simulink model "fec_ber_hw"  (R2020b)
settings: Solver=FixedStepDiscrete  StartTime=0.0  StopTime=T/2  RelTol=1e-3
values from neighbouring files (symbols this model uses):
  aximm_awgn_reset = 0    [setup.m]
  aximm_bit_count_reset = 0    [setup.m]
  aximm_bits = n_blocks * k    (= 3200)    [setup.m]
  aximm_ctrl_word_dec = 0    [setup.m]
  aximm_ctrl_word_enc = 0    [setup.m]
  aximm_enable = 1    [setup.m]
  aximm_length = k * n_blocks    (= 3200)    [setup.m]
  aximm_length_dec = n    (= 160)    [setup.m]
  aximm_length_enc = k    (= 80)    [setup.m]
  aximm_llr_mag_reset = 0    [setup.m]
  aximm_llr_scale = (1/noise_var) * llr_scale    (= 1000)    [setup.m]
  aximm_load_dec = 1    [setup.m]
  aximm_load_enc = 1    [setup.m]
  aximm_noise_std = sqrt(noise_var)    [setup.m]
  aximm_reset = 0    [setup.m]
  d = sqrt(-2*log([0:1/4095:1]))    [setup.m]
  fs = 160e6    (= 160000000)    [setup.m]
  llr_scale = 7.75/7.75    (= 1)    [setup.m]
libraries: simulink x450, hdlsllib x190, commseqgen3 x20, dspsigops x17, lib_rfsoc_fec x5, commblkcod2 x3
(part 1 of 22)
settings Model: SimulationMode=accelerator  Creator=ckb13136  LastModifiedBy=ckb13136
settings OptimizationCC: BlockReduction=off  ConditionallyExecuteInputs=off  DefaultParameterBehavior=Inlined
settings DebuggingCC: AlgebraicLoopMsg=error  SingleTaskRateTransMsg=error
settings HardwareCC: ProdBitPerPointer=32  ProdBitPerSizeT=32  ProdBitPerPtrDiffT=32  ProdLargestAtomicFloat=None  ProdIntDivRoundTo=Undefined  ProdEndianess=Unspecified  ProdWordSize=32  ProdHWDeviceType=ASIC/FPGA->ASIC/FPGA  TargetBitPerPointer=64  TargetBitPerSizeT=64  TargetBitPerPtrDiffT=64  TargetLongLongMode=on  TargetIntDivRoundTo=Zero  TargetEndianess=LittleEndian  TargetWordSize=64  TargetHWDeviceType=Custom Processor->MATLAB Host Computer  ProdEqTarget=off

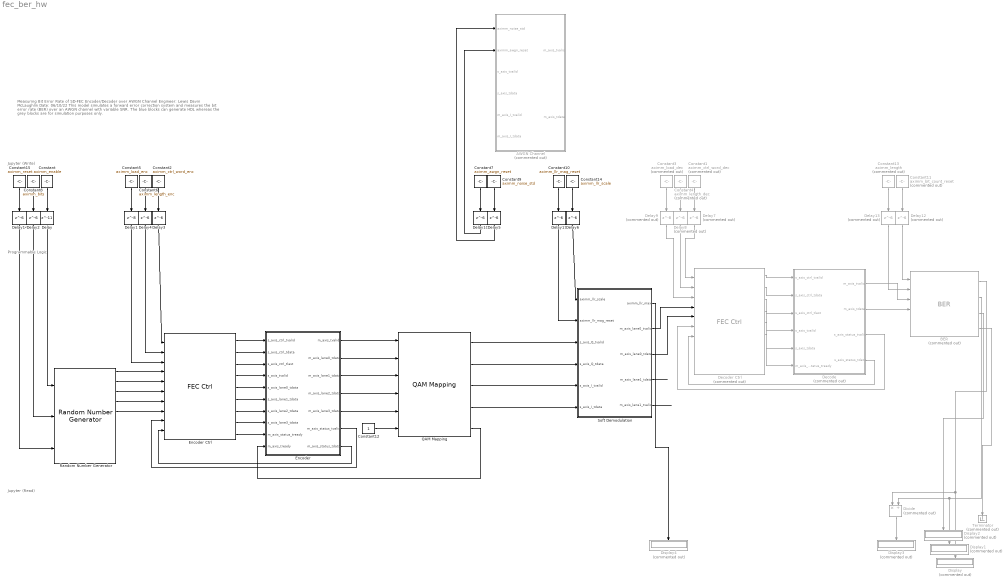
== system fec_ber_hw ==
  note: Measuring Bit Error Rate of SD-FEC Encoder/Decoder over AWGN Channel
      | Engineer: Lewis Davin McLaughlin
      | Date: 06/10/22
      |
      | This model simulates a forward error correction system and measures the bit error rate (BER) over an AWGN channel with variable SNR. The blue blocks can generate HDL whereas the grey blocks are for simulation purposes only.
  note: Jupyter (Write)
  note: Programmable Logic
  note: Jupyter (Read)
  AWGN Channel : Subsystem  Commented=on  AncestorBlock=lib_rfsoc_fec/AWGN Channel  TreatAsAtomicUnit=on
  BER : lib_rfsoc_fec/BER  Commented=on  SystemSampleTime=-1  VariantActivationTime=update diagram  Latency=0  AutoFrameSizeCalculation=off
  Constant : Constant  Value=aximm_enable  OutDataTypeStr=uint32  SampleTime=1/fs
  Constant1 : Constant  Commented=on  Value=aximm_ctrl_word_dec  OutDataTypeStr=uint32  SampleTime=1/(fs*16)
  Constant10 : Constant  Value=aximm_llr_mag_reset  OutDataTypeStr=uint32  SampleTime=1/(fs*2)
  Constant11 : Constant  Commented=on  Value=aximm_bit_count_reset  OutDataTypeStr=uint32  SampleTime=1/(fs*16)
  Constant12 : Constant  OutDataTypeStr=boolean  SampleTime=1/(2*fs)
  Constant13 : Constant  Commented=on  Value=aximm_length  OutDataTypeStr=uint32  SampleTime=1/(fs*16)
  Constant14 : Constant  Value=aximm_llr_scale  OutDataTypeStr=fixdt(0,32,22)  SampleTime=1/(fs*2)
  Constant15 : Constant  Value=aximm_reset  OutDataTypeStr=uint32  SampleTime=1/fs
  Constant2 : Constant  Value=aximm_ctrl_word_enc  OutDataTypeStr=uint32  SampleTime=1/fs
  Constant3 : Constant  Commented=on  Value=aximm_load_dec  OutDataTypeStr=uint32  SampleTime=1/(fs*16)
  Constant4 : Constant  Commented=on  Value=aximm_length_dec  OutDataTypeStr=uint32  SampleTime=1/(fs*16)
  Constant5 : Constant  Value=aximm_load_enc  OutDataTypeStr=uint32  SampleTime=1/fs
  Constant6 : Constant  Value=aximm_length_enc  OutDataTypeStr=uint32  SampleTime=1/fs
  Constant7 : Constant  Value=aximm_awgn_reset  OutDataTypeStr=uint32  SampleTime=1/(fs*2)
  Constant8 : Constant  Value=aximm_bits  OutDataTypeStr=uint32  SampleTime=1/fs
  Constant9 : Constant  Value=aximm_noise_std  OutDataTypeStr=fixdt(0,32,30)  SampleTime=1/(fs*2)
  Decode : Subsystem  Commented=on
  Decoder Ctrl : lib_rfsoc_fec/FEC Ctrl  Commented=on  SystemSampleTime=-1  VariantActivationTime=update diagram  Latency=0  AutoFrameSizeCalculation=off
  Delay : Delay  DelayLength=11
  Delay1 : Delay  DelayLength=8
  Delay{2..6,10..11,14} (8 alike) : Delay  DelayLength=6
  Delay{7..8,12..13} (4 alike) : Delay  Commented=on  DelayLength=6
  Delay9 : Delay  Commented=on  DelayLength=8
  Display{,1..4} (5 alike) : Display  Commented=on
  Divide : Product  Commented=on  Inputs=*/
  Encoder : Subsystem
  Encoder Ctrl : lib_rfsoc_fec/FEC Ctrl  SystemSampleTime=-1  VariantActivationTime=update diagram  Latency=0  AutoFrameSizeCalculation=off
  QAM Mapping : lib_rfsoc_fec/QAM Mapping  SystemSampleTime=-1  VariantActivationTime=update diagram  Latency=0  AutoFrameSizeCalculation=off
  Random Number Generator : lib_rfsoc_fec/Random Number Generator  SystemSampleTime=-1  VariantActivationTime=update diagram  Latency=0  AutoFrameSizeCalculation=off
  Soft Demodulation : Subsystem  AncestorBlock=lib_rfsoc_fec/Soft Demodulation  TreatAsAtomicUnit=on
  Terminator : Terminator  Commented=on
  wires:
  BER/3 -> Display2/1
  Decode/4(s_axis_status_tdata) -> Decoder Ctrl/7
  Soft Demodulation/1(aximm_llr_max) -> Display4/1
  Constant6/1 -> Delay4/1
  Constant3/1 -> Delay9/1
  Decode/3(s_axis_status_tvalid) -> Decoder Ctrl/6
  Constant7/1 -> Delay10/1
  Encoder Ctrl/2 -> Encoder/2(s_axis_ctrl_tdata)
  Decoder Ctrl/6 -> Decode/6(m_axis_status_tready)
  Constant12/1 -> QAM Mapping/6
  Constant4/1 -> Delay8/1
  Encoder Ctrl/6 -> Encoder/6(s_axis_lane1_tdata)
  Constant/1 -> Delay/1
  Delay11/1 -> Soft Demodulation/2(aximm_llr_mag_reset)
  Constant10/1 -> Delay11/1
  Delay9/1 -> Decoder Ctrl/3
  Delay10/1 -> AWGN Channel/2(aximm_awgn_reset)
  Delay/1 -> Random Number Generator/1
  Delay4/1 -> Encoder Ctrl/2
  Delay2/1 -> Random Number Generator/2
  BER/1 -> Divide/1, Display/1
  Soft Demodulation/2(m_axis_lane0_tvalid) -> Decoder Ctrl/4
  Delay12/1 -> BER/1
  Constant11/1 -> Delay12/1
  BER/2 -> Divide/2, Display1/1
  Encoder Ctrl/5 -> Encoder/5(s_axis_lane0_tdata)
  Decoder Ctrl/4 -> Decode/4(s_axis_tvalid)
  Delay8/1 -> Decoder Ctrl/2
  Constant2/1 -> Delay3/1
  Delay7/1 -> Decoder Ctrl/1
  Constant9/1 -> Delay5/1
  Decode/1(m_axis_tvalid) -> BER/3
  Delay1/1 -> Encoder Ctrl/3
  Delay3/1 -> Encoder Ctrl/1
  Decode/2(m_axis_tdata) -> BER/4
  Decoder Ctrl/2 -> Decode/2(s_axis_ctrl_tdata)
  Encoder Ctrl/3 -> Encoder/3(s_axis_ctrl_tlast)
  Decoder Ctrl/3 -> Decode/3(s_axis_ctrl_tlast)
  Divide/1 -> Display3/1
  Encoder/1(m_axis_tvalid) -> QAM Mapping/1
  Delay6/1 -> Soft Demodulation/1(aximm_llr_scale)
  Encoder Ctrl/4 -> Encoder/4(s_axis_tvalid)
  Encoder/7(m_axis_status_tdata) -> Encoder Ctrl/10
  Delay5/1 -> AWGN Channel/1(aximm_noise_std)
  Encoder/2(m_axis_lane0_tdata) -> QAM Mapping/2
  Encoder/6(m_axis_status_tvalid) -> Encoder Ctrl/9
  Decoder Ctrl/1 -> Decode/1(s_axis_ctrl_tvalid)
  Constant14/1 -> Delay6/1
  Decoder Ctrl/5 -> Decode/5(s_axis_tdata)
  Constant8/1 -> Delay2/1
  Encoder Ctrl/1 -> Encoder/1(s_axis_ctrl_tvalid)
  Constant1/1 -> Delay7/1
  Soft Demodulation/3(m_axis_lane0_tdata) -> Decoder Ctrl/5
  Constant5/1 -> Delay1/1
  BER/4 -> Terminator/1
  Constant13/1 -> Delay13/1
  Delay13/1 -> BER/2
  Delay14/1 -> Random Number Generator/3
  Constant15/1 -> Delay14/1
  QAM Mapping/5 -> Encoder/10(m_axis_tready)
  Random Number Generator/3 -> Encoder Ctrl/6
  Random Number Generator/4 -> Encoder Ctrl/7
  Random Number Generator/2 -> Encoder Ctrl/5
  Random Number Generator/1 -> Encoder Ctrl/4
  Random Number Generator/5 -> Encoder Ctrl/8
  Encoder Ctrl/7 -> Encoder/7(s_axis_lane2_tdata)
  Encoder Ctrl/8 -> Encoder/8(s_axis_lane3_tdata)
  Encoder Ctrl/9 -> Encoder/9(m_axis_status_tready)
  Encoder/3(m_axis_lane1_tdata) -> QAM Mapping/3
  Encoder/4(m_axis_lane2_tdata) -> QAM Mapping/4
  Encoder/5(m_axis_lane3_tdata) -> QAM Mapping/5
  QAM Mapping/1 -> Soft Demodulation/3(s_axis_Q_tvalid)
  QAM Mapping/2 -> Soft Demodulation/4(s_axis_Q_tdata)
  QAM Mapping/3 -> Soft Demodulation/5(s_axis_I_tvalid)
  QAM Mapping/4 -> Soft Demodulation/6(s_axis_I_tdata)
  Soft Demodulation/4(m_axis_lane1_tdata) -> ?
  Soft Demodulation/5(m_axis_lane1_tvalid) -> ?

== system fec_ber_hw/AWGN Channel ==
  aximm_noise_std : Inport
  aximm_awgn_reset : Inport  Port=2
  s_axis_tvalid : Inport  Port=3
  s_axis_tdata : Inport  Port=4
  m_axis_I_tvalid : Inport  Port=5
  m_axis_I_tdata : Inport  Port=6
  AWGN Generator : Subsystem
  Add : Sum  OutDataTypeStr=fixdt(1,16,11)  SaturateOnIntegerOverflow=on
  Bit Concat : hdlsllib/Logic and Bit Operations/Bit Concat  numInputs=2
  Bit Slice : hdlsllib/Logic and Bit Operations/Bit Slice  lidx=3  ridx=0
      settings: SourceProductBaseCode=SL
  Bit Slice1 : hdlsllib/Logic and Bit Operations/Bit Slice  lidx=7  ridx=4
      settings: SourceProductBaseCode=SL
  Cast To Boolean : DataTypeConversion  OutDataTypeStr=boolean
  Complex to Real-Imag : ComplexToRealImag
  Data Type Conversion : DataTypeConversion  OutDataTypeStr=fixdt(1,4,0)  ConvertRealWorld=Stored Integer (SI)
  Data Type Conversion1 : DataTypeConversion  OutDataTypeStr=fixdt(1,4,0)  ConvertRealWorld=Stored Integer (SI)
  Delay{,1..5} (6 alike) : Delay
  Downsample{,1..3} (4 alike) : DownSample  N=4  RateOptions=Allow multirate processing
  Real-Imag to Complex : RealImagToComplex
  Repeat : dspsigops/Repeat  N=4  InputProcessing=Columns as channels (frame based)  RateOptions=Allow multirate processing  ic=0  mode=Unused parameter value
      settings: SourceProductName=DSP System Toolbox
  Repeat1 : dspsigops/Repeat  N=4  InputProcessing=Columns as channels (frame based)  RateOptions=Allow multirate processing  ic=0  mode=Unused parameter value
      settings: SourceProductName=DSP System Toolbox
  sample_and_hold : Subsystem
  m_axis_tvalid : Outport
  m_axis_tdata : Outport  Port=2
  wires:
  Cast To Boolean/1 -> Downsample3/1
  aximm_awgn_reset/1 -> Cast To Boolean/1
  Downsample3/1 -> Delay5/1
  Complex to Real-Imag/2 -> Bit Concat/2
  Complex to Real-Imag/1 -> Bit Concat/1
  Bit Concat/1 -> Delay4/1
  Add/1 -> Complex to Real-Imag/1
  Real-Imag to Complex/1 -> Add/1
  Data Type Conversion1/1 -> Real-Imag to Complex/2
  Data Type Conversion/1 -> Real-Imag to Complex/1
  Bit Slice/1 -> Data Type Conversion1/1
  Bit Slice1/1 -> Data Type Conversion/1
  Delay4/1 -> Repeat1/1
  Delay3/1 -> Repeat/1
  Repeat/1 -> m_axis_tvalid/1
  Repeat1/1 -> m_axis_tdata/1
  Delay1/1 -> Bit Slice/1, Bit Slice1/1
  s_axis_tdata/1 -> sample_and_hold/2(data_in)
  s_axis_tvalid/1 -> sample_and_hold/1(valid_in)
  sample_and_hold/2(" data_out") -> Downsample/1
  Delay/1 -> Delay3/1
  Downsample/1 -> Delay1/1
  Downsample1/1 -> Delay/1
  sample_and_hold/1(" valid_out") -> Downsample1/1
  Delay5/1 -> AWGN Generator/2(reset)
  Downsample2/1 -> Delay2/1
  Delay2/1 -> AWGN Generator/1(noise_std)
  aximm_noise_std/1 -> Downsample2/1
  AWGN Generator/1(awgn) -> Add/2

== system fec_ber_hw/Decode ==
  s_axis_ctrl_tvalid : Inport
  s_axis_ctrl_tdata : Inport  Port=2
  s_axis_ctrl_tlast : Inport  Port=3
  s_axis_tvalid : Inport  Port=4
  s_axis_tdata : Inport  Port=5
  m_axis_status_tready : Inport  Port=6
  Bit Concat{,1..3} (4 alike) : hdlsllib/Logic and Bit Operations/Bit Concat  Commented=on  numInputs=2
  Bit Slice : hdlsllib/Logic and Bit Operations/Bit Slice  lidx=5  ridx=0
      settings: SourceProductBaseCode=SL
  Cast To Double : DataTypeConversion  OutDataTypeStr=double
  Cast To Double1 : DataTypeConversion  OutDataTypeStr=double
  Constant3 : Constant  Value=0  OutDataTypeStr=uint32  SampleTime=1/(16*fs)
  Constant4 : Constant  Value=0  OutDataTypeStr=boolean  SampleTime=1/(16*fs)
  Data Type Conversion : DataTypeConversion  OutDataTypeStr=fixdt(1,6,2)  ConvertRealWorld=Stored Integer (SI)
  Data Type Conversion1 : DataTypeConversion  OutDataTypeStr=fixdt(0,128,0)
  Delay : Delay  DelayLength=160
  Delay1 : Delay  DelayLength=1
  Downsample2 : DownSample  N=160  RateOptions=Allow multirate processing
  Downsample3 : DownSample  N=160  RateOptions=Allow multirate processing
  Gain : Gain  Gain=1/llr_scale
  LDPC Decoder : commblkcod2/LDPC Decoder  ParityCheckMat=parity_sparse  OutputFmt=Information part  DecisionType=Hard decision  OutputDataType=boolean  NumIter=50  DoParityCheck=off  OutputNumIter=off  OutputFinalChecks=off
      settings: SourceProductBaseCode=CM
  MATLAB Function : MATLAB Function  TreatAsAtomicUnit=on
  MATLAB Function1 : MATLAB Function  TreatAsAtomicUnit=on
  MATLAB Function5 : MATLAB Function  Commented=on  TreatAsAtomicUnit=on
  NOT1 : Logic  Operator=NOT  IconShape=distinctive  AllPortsSameDT=off  OutDataTypeStr=boolean
  NOT2 : Logic  Commented=on  Operator=NOT  IconShape=distinctive  AllPortsSameDT=off  OutDataTypeStr=boolean
  Rate Transition : RateTransition
  Repeat : dspsigops/Repeat  N=10  InputProcessing=Columns as channels (frame based)  RateOptions=Allow multirate processing  ic=0  mode=Unused parameter value
      settings: SourceProductName=DSP System Toolbox
  Subsystem : Subsystem  Commented=on
  Terminator{,1..3} (4 alike) : Terminator
  Upsample : dspsigops/Upsample  N=16  phase=0  RateOptions=Allow multirate processing  ic=0  mode=Unused parameter value
  Upsample1 : dspsigops/Upsample  N=16  phase=0  RateOptions=Allow multirate processing  ic=0  mode=Unused parameter value
  m_axis_tvalid : Outport
  m_axis_tdata : Outport  Port=2
  s_axis_status_tvalid : Outport  Port=3
  s_axis_status_tdata : Outport  Port=4
  wires:
  s_axis_tvalid/1 -> Delay/1, MATLAB Function/1(valid)
  MATLAB Function/1(frame) -> Downsample2/1
  Data Type Conversion/1 -> Gain/1
  Bit Slice/1 -> Data Type Conversion/1
  Cast To Double/1 -> MATLAB Function/2(sample)
  Gain/1 -> Cast To Double/1
  s_axis_tdata/1 -> Bit Slice/1
  Downsample3/1 -> Delay1/1
  s_axis_ctrl_tvalid/1 -> Terminator/1
  s_axis_ctrl_tdata/1 -> Terminator1/1
  s_axis_ctrl_tlast/1 -> Terminator2/1
  m_axis_status_tready/1 -> Terminator3/1
  Constant4/1 -> s_axis_status_tvalid/1
  Constant3/1 -> s_axis_status_tdata/1
  Downsample2/1 -> LDPC Decoder/1
  Delay/1 -> Downsample3/1
  LDPC Decoder/1 -> NOT1/1
  NOT1/1 -> Cast To Double1/1
  MATLAB Function1/1(uint8) -> Upsample1/1
  Upsample/1 -> m_axis_tvalid/1
  Upsample1/1 -> Data Type Conversion1/1
  Cast To Double1/1 -> Rate Transition/1
  Rate Transition/1 -> MATLAB Function1/2(frame)
  Data Type Conversion1/1 -> m_axis_tdata/1
  Repeat/1 -> Upsample/1, MATLAB Function1/1(valid)
  Delay1/1 -> Repeat/1
  Bit Concat3/1 -> ?
  MATLAB Function5/1(tvalid) -> ?
  Bit Concat1/1 -> ?
  Bit Concat2/1 -> ?
  Bit Concat/1 -> ?
  MATLAB Function5/2(lane_0) -> Bit Concat/2
  MATLAB Function5/7(lane_5) -> Bit Concat2/1
  MATLAB Function5/9(lane_7) -> Bit Concat3/1
  NOT2/1 -> MATLAB Function5/3(frame)
  MATLAB Function5/6(lane_4) -> Bit Concat2/2
  Subsystem/1(Out1) -> NOT2/1
  MATLAB Function5/3(lane_1) -> Bit Concat/1
  MATLAB Function5/5(lane_3) -> Bit Concat1/1
  MATLAB Function5/8(lane_6) -> Bit Concat3/2
  MATLAB Function5/4(lane_2) -> Bit Concat1/2

== system fec_ber_hw/Encoder ==
  s_axis_ctrl_tvalid : Inport
  s_axis_ctrl_tdata : Inport  Port=2
  s_axis_ctrl_tlast : Inport  Port=3
  s_axis_tvalid : Inport  Port=4
  s_axis_lane0_tdata : Inport  Port=5
  s_axis_lane1_tdata : Inport  Port=6
  s_axis_lane2_tdata : Inport  Port=7
  s_axis_lane3_tdata : Inport  Port=8
  m_axis_status_tready : Inport  Port=9
  m_axis_tready : Inport  Port=10
  Bit Concat{4..7} (4 alike) : hdlsllib/Logic and Bit Operations/Bit Concat  numInputs=2
  Bit Slice{,2,4,6} (4 alike) : hdlsllib/Logic and Bit Operations/Bit Slice  lidx=63  ridx=0
      settings: SourceProductBaseCode=SL
  Bit Slice{1,3,5,7} (4 alike) : hdlsllib/Logic and Bit Operations/Bit Slice  lidx=127  ridx=64
      settings: SourceProductBaseCode=SL
  Constant1 : Constant  Value=aximm_bits * 2  OutDataTypeStr=uint32  SampleTime=1/(8*fs)
  Constant3 : Constant  Value=0  OutDataTypeStr=uint32  SampleTime=1/fs
  Constant4 : Constant  Value=0  OutDataTypeStr=boolean  SampleTime=1/fs
  Constant8 : Constant  Value=aximm_bits  OutDataTypeStr=uint32  SampleTime=1/(8*fs)
  Downsample{4..8} (5 alike) : DownSample  N=4  RateOptions=Allow multirate processing
  Encode : Subsystem
  MATLAB Function3 : MATLAB Function  TreatAsAtomicUnit=on
  MATLAB Function4 : MATLAB Function  TreatAsAtomicUnit=on
  Repeat{,2..4} (4 alike) : dspsigops/Repeat  N=8  InputProcessing=Columns as channels (frame based)  RateOptions=Allow multirate processing  ic=0  mode=Unused parameter value
      settings: SourceProductName=DSP System Toolbox
  Terminator{,1..4} (5 alike) : Terminator
  Upsample2 : dspsigops/Upsample  N=8  phase=0  RateOptions=Allow multirate processing  ic=0  mode=Unused parameter value
  sample_and_hold : Subsystem
  m_axis_tvalid : Outport
  m_axis_lane0_tdata : Outport  Port=2
  m_axis_lane1_tdata : Outport  Port=3
  m_axis_lane2_tdata : Outport  Port=4
  m_axis_lane3_tdata : Outport  Port=5
  m_axis_status_tvalid : Outport  Port=6
  m_axis_status_tdata : Outport  Port=7
  wires:
  Constant3/1 -> m_axis_status_tdata/1
  Constant4/1 -> m_axis_status_tvalid/1
  s_axis_ctrl_tvalid/1 -> Terminator/1
  s_axis_ctrl_tdata/1 -> Terminator1/1
  s_axis_ctrl_tlast/1 -> Terminator2/1
  m_axis_status_tready/1 -> Terminator3/1
  m_axis_tready/1 -> Terminator4/1
  MATLAB Function3/2(frame_out) -> Encode/1(frame_out)
  MATLAB Function3/1(valid_out) -> MATLAB Function4/2(valid), Encode/Enable
  s_axis_tvalid/1 -> Upsample2/1
  s_axis_lane0_tdata/1 -> Repeat/1
  s_axis_lane1_tdata/1 -> Repeat2/1
  s_axis_lane2_tdata/1 -> Repeat3/1
  s_axis_lane3_tdata/1 -> Repeat4/1
  Upsample2/1 -> MATLAB Function3/2(valid)
  Repeat/1 -> Bit Slice1/1, Bit Slice/1
  Bit Slice/1 -> MATLAB Function3/3(lane_0)
  Bit Slice1/1 -> MATLAB Function3/4(lane_1)
  Repeat2/1 -> Bit Slice2/1, Bit Slice3/1
  Repeat3/1 -> Bit Slice4/1, Bit Slice5/1
  Repeat4/1 -> Bit Slice6/1, Bit Slice7/1
  Bit Slice2/1 -> MATLAB Function3/5(lane_2)
  Bit Slice3/1 -> MATLAB Function3/6(lane_3)
  Bit Slice4/1 -> MATLAB Function3/7(lane_4)
  Bit Slice5/1 -> MATLAB Function3/8(lane_5)
  Bit Slice6/1 -> MATLAB Function3/9(lane_6)
  Bit Slice7/1 -> MATLAB Function3/10(lane_7)
  Constant8/1 -> MATLAB Function3/1(bits)
  Encode/1(frame) -> MATLAB Function4/3(frame)
  Bit Concat7/1 -> sample_and_hold/5(s_axis_lane3_tdata)
  Bit Concat6/1 -> sample_and_hold/4(s_axis_lane2_tdata)
  Bit Concat5/1 -> sample_and_hold/3(s_axis_lane1_tdata)
  Bit Concat4/1 -> sample_and_hold/2(s_axis_lane0_tdata)
  MATLAB Function4/9(lane_7) -> Bit Concat7/1
  MATLAB Function4/8(lane_6) -> Bit Concat7/2
  MATLAB Function4/7(lane_5) -> Bit Concat6/1
  MATLAB Function4/6(lane_4) -> Bit Concat6/2
  MATLAB Function4/5(lane_3) -> Bit Concat5/1
  MATLAB Function4/4(lane_2) -> Bit Concat5/2
  MATLAB Function4/3(lane_1) -> Bit Concat4/1
  MATLAB Function4/2(lane_0) -> Bit Concat4/2
  MATLAB Function4/1(tvalid) -> sample_and_hold/1(s_axis_tvalid)
  sample_and_hold/1(" valid_out") -> Downsample4/1
  sample_and_hold/2(" m_axis_lane0_tdata") -> Downsample5/1
  sample_and_hold/3(" m_axis_lane1_tdata") -> Downsample6/1
  sample_and_hold/4(" m_axis_lane2_tdata") -> Downsample7/1
  sample_and_hold/5(" m_axis_lane3_tdata") -> Downsample8/1
  Downsample4/1 -> m_axis_tvalid/1
  Downsample5/1 -> m_axis_lane0_tdata/1
  Downsample6/1 -> m_axis_lane1_tdata/1
  Downsample7/1 -> m_axis_lane2_tdata/1
  Downsample8/1 -> m_axis_lane3_tdata/1
  Constant1/1 -> MATLAB Function4/1(bits)

== system fec_ber_hw/Soft Demodulation ==
  aximm_llr_scale : Inport
  aximm_llr_mag_reset : Inport  Port=2
  s_axis_Q_tvalid : Inport  Port=3
  s_axis_Q_tdata : Inport  Port=4
  s_axis_I_tvalid : Inport  Port=5
  s_axis_I_tdata : Inport  Port=6
  Bit Slice1 : hdlsllib/Logic and Bit Operations/Bit Slice  lidx=95  ridx=48
      settings: SourceProductBaseCode=SL
  Bit Slice2 : hdlsllib/Logic and Bit Operations/Bit Slice  lidx=47  ridx=0
      settings: SourceProductBaseCode=SL
  Bit Slice3 : hdlsllib/Logic and Bit Operations/Bit Slice  lidx=47  ridx=0
      settings: SourceProductBaseCode=SL
  Bit Slice4 : hdlsllib/Logic and Bit Operations/Bit Slice  lidx=95  ridx=48
      settings: SourceProductBaseCode=SL
  Cast To Boolean : DataTypeConversion  Commented=on  OutDataTypeStr=boolean
  MATLAB Function : MATLAB Function  Commented=on  TreatAsAtomicUnit=on
  SSR Soft Demodulation Lane 0 : Subsystem  mask{ssr=16}
      mask init:
      | top_block = gcb;
      | 
      | block_names = find_system(top_block, 'LookUnderMasks','on', 'SearchDepth','1');
      | 
      | in_valid = sprintf('%s/valid', top_block);
      | in_real = sprintf('%s/real', top_block);
      | in_imag = sprintf('%s/imag', top_block);
      | in_scale = sprintf('%s/scale', top_block);
      | out_llr = sprintf('%s/llr', top_block);
      | soft_demod_block = sprintf('%s/Soft Demodulation 0', top_block);
      | 
      | keep_blocks = {top_block,in_valid,in_real,in_imag,in_scale,soft_demod_block,out_llr};
      | 
      | for i = 1:length(block_names)
      |     if ~ismember(block_names{i}, keep_blocks)
      |         delete_block(block_names{i});
      |     end
      | end
      | delete_line(find_system(top_block,'LookUnderMasks', 'all','SearchDepth', '1', 'FindAll','on','type','line'));
      | 
      | % Add Soft Demodulation Blocks
      | pos = get_param(soft_demod_block, 'position');
      | new_pos = pos;
      | for i = 1:ssr-1
      |     new_block = sprintf('%s%d', soft_demod_block(1:end-1), i);
      |     add_block(soft_demod_block, new_block);
      |     new_pos = pos + ([0 150 0 150] * i);
      |     set_param(new_block, 'position', new_pos);
      |     set_param(new_block, 'n', num2str(i+1));
      | end
      | 
      | % Add the Bit Concat
      | concat_block = sprintf('%s/concat', top_block);
      | add_block('hdlsllib/Logic and Bit Operations/Bit Concat', concat_block);
      | set_param(concat_block, 'numInputs', num2str(ssr));
      | concat_position = new_pos + [275 0 175 0];
      | concat_position(2) = pos(2);
      | set_param(concat_block, 'position', concat_position);
      | 
      | % Reposition Output
      | out_position = get_param(out_llr, 'position');
      | height = out_position(4) - out_position(2);
      | width = out_position(3) - out_position(1);
      | middle_h = (concat_position(4) - concat_position(2))/2 + concat_position(2);
      | out_position = [concat_position(1) + 175, middle_h - height/2, concat_position(1) + 175 + width, middle_h + height/2];
      | set_param(out_llr, 'position', out_position);
      | 
      | % Connect Ports
      | for i = 1:ssr
      |     add_line(top_block,'valid/1',sprintf('Soft Demodulation %d/1',i-1));
      |     add_line(top_block,'real/1',sprintf('Soft Demodulation %d/2',i-1));
      |     add_line(top_block,'imag/1',sprintf('Soft Demodulation %d/3',i-1));
      |     add_line(top_block,'scale/1',sprintf('Soft Demodulation %d/4',i-1));
      |     
      |     add_line(top_block,sprintf('Soft Demodulation %d/1',i-1),sprintf('concat/%d', i));
      | end
      | add_line(top_block,'concat/1','llr/1');
  SSR Soft Demodulation Lane 1 : Subsystem  mask{ssr=16}
      mask init: same as fec_ber_hw/Soft Demodulation/SSR Soft Demodulation Lane 0
  aximm_llr_max : Outport
  m_axis_lane0_tvalid : Outport  Port=2
  m_axis_lane0_tdata : Outport  Port=3
  m_axis_lane1_tdata : Outport  Port=4
  m_axis_lane1_tvalid : Outport  Port=5
  wires:
  Cast To Boolean/1 -> MATLAB Function/2(reset)
  aximm_llr_mag_reset/1 -> Cast To Boolean/1
  MATLAB Function/1(y) -> aximm_llr_max/1
  aximm_llr_scale/1 -> SSR Soft Demodulation Lane 1/4(scale), SSR Soft Demodulation Lane 0/4(scale)
  Bit Slice2/1 -> SSR Soft Demodulation Lane 0/2(real)
  Bit Slice3/1 -> SSR Soft Demodulation Lane 0/3(imag)
  s_axis_I_tdata/1 -> Bit Slice1/1, Bit Slice2/1
  s_axis_Q_tdata/1 -> Bit Slice4/1, Bit Slice3/1
  s_axis_Q_tvalid/1 -> SSR Soft Demodulation Lane 1/1(valid), SSR Soft Demodulation Lane 0/1(valid)
  Bit Slice1/1 -> SSR Soft Demodulation Lane 1/2(real)
  Bit Slice4/1 -> SSR Soft Demodulation Lane 1/3(imag)
  SSR Soft Demodulation Lane 0/1(llr) -> m_axis_lane0_tdata/1
  s_axis_I_tvalid/1 -> m_axis_lane1_tvalid/1, m_axis_lane0_tvalid/1
  SSR Soft Demodulation Lane 1/1(llr) -> m_axis_lane1_tdata/1

== system fec_ber_hw/AWGN Channel/AWGN Generator ==
  noise_std : Inport
  reset : Inport  Port=2
  1-D Lookup Table : Lookup_n-D  NumberOfTableDimensions=1  BreakpointsForDimension1=[0:4095]  BreakpointsForDimension1DataTypeStr=fixdt(0,12,0)  IndexSearchMethod=Evenly spaced points  Table=d  InterpMethod=Flat  ExtrapMethod=Clip  DiagnosticForOutOfRangeInput=Error  InternalRulePriority=Speed  OutDataTypeStr=fixdt(1,18,14)  RndMeth=Simplest  InputSameDT=on
  Cosine Lookup : Lookup_n-D  NumberOfTableDimensions=1  BreakpointsForDimension1=[0:255]  IndexSearchMethod=Evenly spaced points  Table=cos([0:255]*2*pi/256)  InterpMethod=Flat  ExtrapMethod=Clip  DiagnosticForOutOfRangeInput=Error  UseLastTableValue=on  OutDataTypeStr=fixdt(1,16,14)  RndMeth=Simplest  InputSameDT=on
  Data Type Conversion : DataTypeConversion  OutDataTypeStr=fixdt(0,16,14)  RndMeth=Round  SaturateOnIntegerOverflow=on
  Gain : Gain  Gain=0.7  OutDataTypeStr=fixdt(1,15,11)  RndMeth=Nearest  SaturateOnIntegerOverflow=on
  Product : Product  OutDataTypeStr=fixdt(1,17,14)  RndMeth=Round  SaturateOnIntegerOverflow=on
  Product1 : Product  OutDataTypeStr=fixdt(1,17,14)  RndMeth=Round  SaturateOnIntegerOverflow=on
  Product3 : Product  OutDataTypeStr=fixdt(1,18,14)  RndMeth=Round
  Real-Imag to Complex1 : RealImagToComplex
  Sine Lookup : Lookup_n-D  NumberOfTableDimensions=1  BreakpointsForDimension1=[0:255]  IndexSearchMethod=Evenly spaced points  Table=sin([0:255]*2*pi/256)  InterpMethod=Flat  ExtrapMethod=Clip  DiagnosticForOutOfRangeInput=Error  UseLastTableValue=on  OutDataTypeStr=fixdt(1,16,14)  RndMeth=Simplest  InputSameDT=on
  Subsystem3 : Subsystem
  awgn : Outport
  wires:
  Data Type Conversion/1 -> Product3/1
  Real-Imag to Complex1/1 -> Product3/2
  Gain/1 -> awgn/1
  Cosine Lookup/1 -> Product1/1
  Subsystem3/1(LFSR_G) -> Sine Lookup/1, Cosine Lookup/1
  1-D Lookup Table/1 -> Product/2, Product1/2
  Subsystem3/2(LFSR_F) -> 1-D Lookup Table/1
  reset/1 -> Subsystem3/1(Reset)
  Sine Lookup/1 -> Product/1
  Product3/1 -> Gain/1
  Product/1 -> Real-Imag to Complex1/2
  Product1/1 -> Real-Imag to Complex1/1
  noise_std/1 -> Data Type Conversion/1

== system fec_ber_hw/AWGN Channel/sample_and_hold ==
  valid_in : Inport
  data_in : Inport  Port=2
  Sample and Hold : dspsigops/Sample and Hold  trig=Rising edge  initCond=0  latchinput=off
  tvalid hold : Subsystem
  " valid_out" : Outport
  " data_out" : Outport  Port=2
  wires:
  Sample and Hold/1 -> " data_out"/1
  data_in/1 -> Sample and Hold/1
  tvalid hold/1(" ") -> " valid_out"/1
  valid_in/1 -> Sample and Hold/Trigger, tvalid hold/1(In1)

== system fec_ber_hw/Decode/Subsystem ==
  In1 : Inport
  Enable : EnablePort
  LDPC Decoder : commblkcod2/LDPC Decoder  ParityCheckMat=parity_sparse  OutputFmt=Information part  DecisionType=Hard decision  OutputDataType=boolean  NumIter=64  DoParityCheck=on  OutputNumIter=off  OutputFinalChecks=off
      settings: SourceProductBaseCode=CM
  Out1 : Outport
  wires:
  LDPC Decoder/1 -> Out1/1
  In1/1 -> LDPC Decoder/1

== system fec_ber_hw/Encoder/Encode ==
  frame_out : Inport
  Enable : EnablePort
  Cast To Boolean1 : DataTypeConversion  OutDataTypeStr=boolean
  Cast To Double : DataTypeConversion  OutDataTypeStr=double
  LDPC Encoder1 : commblkcod2/LDPC Encoder  ParityCheckMat=parity_sparse
      settings: SourceProductBaseCode=CM
  frame : Outport
  wires:
  LDPC Encoder1/1 -> Cast To Boolean1/1
  Cast To Boolean1/1 -> frame/1
  Cast To Double/1 -> LDPC Encoder1/1
  frame_out/1 -> Cast To Double/1

== system fec_ber_hw/Encoder/sample_and_hold ==
  s_axis_tvalid : Inport
  s_axis_lane0_tdata : Inport  Port=2
  s_axis_lane1_tdata : Inport  Port=3
  s_axis_lane2_tdata : Inport  Port=4
  s_axis_lane3_tdata : Inport  Port=5
  Sample and Hold{,1..3} (4 alike) : dspsigops/Sample and Hold  trig=Rising edge  initCond=0  latchinput=off
  tvalid hold : Subsystem
  " valid_out" : Outport
  " m_axis_lane0_tdata" : Outport  Port=2
  " m_axis_lane1_tdata" : Outport  Port=3
  " m_axis_lane2_tdata" : Outport  Port=4
  " m_axis_lane3_tdata" : Outport  Port=5
  wires:
  Sample and Hold/1 -> " m_axis_lane0_tdata"/1
  s_axis_lane0_tdata/1 -> Sample and Hold/1
  tvalid hold/1(" ") -> " valid_out"/1
  s_axis_tvalid/1 -> Sample and Hold1/Trigger, tvalid hold/1(In1), Sample and Hold3/Trigger, Sample and Hold2/Trigger, Sample and Hold/Trigger
  s_axis_lane1_tdata/1 -> Sample and Hold1/1
  s_axis_lane2_tdata/1 -> Sample and Hold2/1
  s_axis_lane3_tdata/1 -> Sample and Hold3/1
  Sample and Hold1/1 -> " m_axis_lane1_tdata"/1
  Sample and Hold2/1 -> " m_axis_lane2_tdata"/1
  Sample and Hold3/1 -> " m_axis_lane3_tdata"/1

== system fec_ber_hw/Soft Demodulation/SSR Soft Demodulation Lane 0 ==
  valid : Inport
  real : Inport  Port=2
  imag : Inport  Port=3
  scale : Inport  Port=4
  Soft Demodulation 0 : Subsystem  mask{w=3, f=0, n=1}
  Soft Demodulation 1 : Subsystem  mask{w=3, f=0, n=2}
  Soft Demodulation 10 : Subsystem  mask{w=3, f=0, n=11}
  Soft Demodulation 11 : Subsystem  mask{w=3, f=0, n=12}
  Soft Demodulation 12 : Subsystem  mask{w=3, f=0, n=13}
  Soft Demodulation 13 : Subsystem  mask{w=3, f=0, n=14}
  Soft Demodulation 14 : Subsystem  mask{w=3, f=0, n=15}
  Soft Demodulation 15 : Subsystem  mask{w=3, f=0, n=16}
  Soft Demodulation 2 : Subsystem  mask{w=3, f=0, n=3}
  Soft Demodulation 3 : Subsystem  mask{w=3, f=0, n=4}
  Soft Demodulation 4 : Subsystem  mask{w=3, f=0, n=5}
  Soft Demodulation 5 : Subsystem  mask{w=3, f=0, n=6}
  Soft Demodulation 6 : Subsystem  mask{w=3, f=0, n=7}
  Soft Demodulation 7 : Subsystem  mask{w=3, f=0, n=8}
  Soft Demodulation 8 : Subsystem  mask{w=3, f=0, n=9}
  Soft Demodulation 9 : Subsystem  mask{w=3, f=0, n=10}
  concat : hdlsllib/Logic and Bit Operations/Bit Concat  numInputs=16
  llr : Outport
  wires:
  valid/1 -> Soft Demodulation 0/1(valid), Soft Demodulation 1/1(valid), Soft Demodulation 2/1(valid), Soft Demodulation 3/1(valid), Soft Demodulation 4/1(valid), Soft Demodulation 5/1(valid), Soft Demodulation 6/1(valid), Soft Demodulation 7/1(valid), Soft Demodulation 8/1(valid), Soft Demodulation 9/1(valid), Soft Demodulation 10/1(valid), Soft Demodulation 11/1(valid), Soft Demodulation 12/1(valid), Soft Demodulation 13/1(valid), Soft Demodulation 14/1(valid), Soft Demodulation 15/1(valid)
  real/1 -> Soft Demodulation 0/2(real), Soft Demodulation 1/2(real), Soft Demodulation 2/2(real), Soft Demodulation 3/2(real), Soft Demodulation 4/2(real), Soft Demodulation 5/2(real), Soft Demodulation 6/2(real), Soft Demodulation 7/2(real), Soft Demodulation 8/2(real), Soft Demodulation 9/2(real), Soft Demodulation 10/2(real), Soft Demodulation 11/2(real), Soft Demodulation 12/2(real), Soft Demodulation 13/2(real), Soft Demodulation 14/2(real), Soft Demodulation 15/2(real)
  imag/1 -> Soft Demodulation 0/3(imag), Soft Demodulation 1/3(imag), Soft Demodulation 2/3(imag), Soft Demodulation 3/3(imag), Soft Demodulation 4/3(imag), Soft Demodulation 5/3(imag), Soft Demodulation 6/3(imag), Soft Demodulation 7/3(imag), Soft Demodulation 8/3(imag), Soft Demodulation 9/3(imag), Soft Demodulation 10/3(imag), Soft Demodulation 11/3(imag), Soft Demodulation 12/3(imag), Soft Demodulation 13/3(imag), Soft Demodulation 14/3(imag), Soft Demodulation 15/3(imag)
  scale/1 -> Soft Demodulation 0/4(LLR Scale), Soft Demodulation 1/4(LLR Scale), Soft Demodulation 2/4(LLR Scale), Soft Demodulation 3/4(LLR Scale), Soft Demodulation 4/4(LLR Scale), Soft Demodulation 5/4(LLR Scale), Soft Demodulation 6/4(LLR Scale), Soft Demodulation 7/4(LLR Scale), Soft Demodulation 8/4(LLR Scale), Soft Demodulation 9/4(LLR Scale), Soft Demodulation 10/4(LLR Scale), Soft Demodulation 11/4(LLR Scale), Soft Demodulation 12/4(LLR Scale), Soft Demodulation 13/4(LLR Scale), Soft Demodulation 14/4(LLR Scale), Soft Demodulation 15/4(LLR Scale)
  Soft Demodulation 0/1(LLR Values) -> concat/1
  Soft Demodulation 1/1(LLR Values) -> concat/2
  Soft Demodulation 2/1(LLR Values) -> concat/3
  Soft Demodulation 3/1(LLR Values) -> concat/4
  Soft Demodulation 4/1(LLR Values) -> concat/5
  Soft Demodulation 5/1(LLR Values) -> concat/6
  Soft Demodulation 6/1(LLR Values) -> concat/7
  Soft Demodulation 7/1(LLR Values) -> concat/8
  Soft Demodulation 8/1(LLR Values) -> concat/9
  Soft Demodulation 9/1(LLR Values) -> concat/10
  Soft Demodulation 10/1(LLR Values) -> concat/11
  Soft Demodulation 11/1(LLR Values) -> concat/12
  Soft Demodulation 12/1(LLR Values) -> concat/13
  Soft Demodulation 13/1(LLR Values) -> concat/14
  Soft Demodulation 14/1(LLR Values) -> concat/15
  Soft Demodulation 15/1(LLR Values) -> concat/16
  concat/1 -> llr/1

== system fec_ber_hw/Soft Demodulation/SSR Soft Demodulation Lane 1 ==
  valid : Inport
  real : Inport  Port=2
  imag : Inport  Port=3
  scale : Inport  Port=4
  Soft Demodulation 0 : Subsystem  mask{w=3, f=0, n=1}
  Soft Demodulation 1 : Subsystem  mask{w=3, f=0, n=2}
  Soft Demodulation 10 : Subsystem  mask{w=3, f=0, n=11}
  Soft Demodulation 11 : Subsystem  mask{w=3, f=0, n=12}
  Soft Demodulation 12 : Subsystem  mask{w=3, f=0, n=13}
  Soft Demodulation 13 : Subsystem  mask{w=3, f=0, n=14}
  Soft Demodulation 14 : Subsystem  mask{w=3, f=0, n=15}
  Soft Demodulation 15 : Subsystem  mask{w=3, f=0, n=16}
  Soft Demodulation 2 : Subsystem  mask{w=3, f=0, n=3}
  Soft Demodulation 3 : Subsystem  mask{w=3, f=0, n=4}
  Soft Demodulation 4 : Subsystem  mask{w=3, f=0, n=5}
  Soft Demodulation 5 : Subsystem  mask{w=3, f=0, n=6}
  Soft Demodulation 6 : Subsystem  mask{w=3, f=0, n=7}
  Soft Demodulation 7 : Subsystem  mask{w=3, f=0, n=8}
  Soft Demodulation 8 : Subsystem  mask{w=3, f=0, n=9}
  Soft Demodulation 9 : Subsystem  mask{w=3, f=0, n=10}
  concat : hdlsllib/Logic and Bit Operations/Bit Concat  numInputs=16
  llr : Outport
  wires:
  valid/1 -> Soft Demodulation 0/1(valid), Soft Demodulation 1/1(valid), Soft Demodulation 2/1(valid), Soft Demodulation 3/1(valid), Soft Demodulation 4/1(valid), Soft Demodulation 5/1(valid), Soft Demodulation 6/1(valid), Soft Demodulation 7/1(valid), Soft Demodulation 8/1(valid), Soft Demodulation 9/1(valid), Soft Demodulation 10/1(valid), Soft Demodulation 11/1(valid), Soft Demodulation 12/1(valid), Soft Demodulation 13/1(valid), Soft Demodulation 14/1(valid), Soft Demodulation 15/1(valid)
  real/1 -> Soft Demodulation 0/2(real), Soft Demodulation 1/2(real), Soft Demodulation 2/2(real), Soft Demodulation 3/2(real), Soft Demodulation 4/2(real), Soft Demodulation 5/2(real), Soft Demodulation 6/2(real), Soft Demodulation 7/2(real), Soft Demodulation 8/2(real), Soft Demodulation 9/2(real), Soft Demodulation 10/2(real), Soft Demodulation 11/2(real), Soft Demodulation 12/2(real), Soft Demodulation 13/2(real), Soft Demodulation 14/2(real), Soft Demodulation 15/2(real)
  imag/1 -> Soft Demodulation 0/3(imag), Soft Demodulation 1/3(imag), Soft Demodulation 2/3(imag), Soft Demodulation 3/3(imag), Soft Demodulation 4/3(imag), Soft Demodulation 5/3(imag), Soft Demodulation 6/3(imag), Soft Demodulation 7/3(imag), Soft Demodulation 8/3(imag), Soft Demodulation 9/3(imag), Soft Demodulation 10/3(imag), Soft Demodulation 11/3(imag), Soft Demodulation 12/3(imag), Soft Demodulation 13/3(imag), Soft Demodulation 14/3(imag), Soft Demodulation 15/3(imag)
  scale/1 -> Soft Demodulation 0/4(LLR Scale), Soft Demodulation 1/4(LLR Scale), Soft Demodulation 2/4(LLR Scale), Soft Demodulation 3/4(LLR Scale), Soft Demodulation 4/4(LLR Scale), Soft Demodulation 5/4(LLR Scale), Soft Demodulation 6/4(LLR Scale), Soft Demodulation 7/4(LLR Scale), Soft Demodulation 8/4(LLR Scale), Soft Demodulation 9/4(LLR Scale), Soft Demodulation 10/4(LLR Scale), Soft Demodulation 11/4(LLR Scale), Soft Demodulation 12/4(LLR Scale), Soft Demodulation 13/4(LLR Scale), Soft Demodulation 14/4(LLR Scale), Soft Demodulation 15/4(LLR Scale)
  Soft Demodulation 0/1(LLR Values) -> concat/1
  Soft Demodulation 1/1(LLR Values) -> concat/2
  Soft Demodulation 2/1(LLR Values) -> concat/3
  Soft Demodulation 3/1(LLR Values) -> concat/4
  Soft Demodulation 4/1(LLR Values) -> concat/5
  Soft Demodulation 5/1(LLR Values) -> concat/6
  Soft Demodulation 6/1(LLR Values) -> concat/7
  Soft Demodulation 7/1(LLR Values) -> concat/8
  Soft Demodulation 8/1(LLR Values) -> concat/9
  Soft Demodulation 9/1(LLR Values) -> concat/10
  Soft Demodulation 10/1(LLR Values) -> concat/11
  Soft Demodulation 11/1(LLR Values) -> concat/12
  Soft Demodulation 12/1(LLR Values) -> concat/13
  Soft Demodulation 13/1(LLR Values) -> concat/14
  Soft Demodulation 14/1(LLR Values) -> concat/15
  Soft Demodulation 15/1(LLR Values) -> concat/16
  concat/1 -> llr/1

== system fec_ber_hw/AWGN Channel/AWGN Generator/Subsystem3 ==
  note: here
  Reset : Inport
  Bit Concat : hdlsllib/Logic and Bit Operations/Bit Concat  numInputs=8
  Bit Concat1 : hdlsllib/Logic and Bit Operations/Bit Concat  numInputs=12
  PN Sequence Generator : commseqgen3/PN Sequence Generator  poly='z^13 + z^12 + z^11 + z^8 + 1'  ini_sta=[0 1 1 0 0 0 0 0 0 1 0 0 0]  outBitMaskSource=Dialog parameter  shift=0  outVarSiz=off  maxOutSizeMode=Dialog parameter  maxOutSize=[10 1]  Ts=-1  sampPerFrame=1  reset=on  bitPackedOutputs=off  outDataType=boolean  numPackedBits=8  bitPackDataSigned=off  bitPackedOutDType=Smallest integer
  PN Sequence Generator1 : commseqgen3/PN Sequence Generator  poly='z^13 + z^12 + z^11 + z^8 + 1'  ini_sta=[0 0 1 1 0 0 0 0 0 0 0 1 1]  outBitMaskSource=Dialog parameter  shift=0  outVarSiz=off  maxOutSizeMode=Dialog parameter  maxOutSize=[10 1]  Ts=-1  sampPerFrame=1  reset=on  bitPackedOutputs=off  outDataType=boolean  numPackedBits=8  bitPackDataSigned=off  bitPackedOutDType=Smallest integer
  PN Sequence Generator10 : commseqgen3/PN Sequence Generator  poly='z^13 + z^12 + z^11 + z^8 + 1'  ini_sta=[1 0 0 0 0 0 1 0 0 0 0 0 1]  outBitMaskSource=Dialog parameter  shift=0  outVarSiz=off  maxOutSizeMode=Dialog parameter  maxOutSize=[10 1]  Ts=-1  sampPerFrame=1  reset=on  bitPackedOutputs=off  outDataType=boolean  numPackedBits=8  bitPackDataSigned=off  bitPackedOutDType=Smallest integer
  PN Sequence Generator11 : commseqgen3/PN Sequence Generator  poly='z^13 + z^12 + z^11 + z^8 + 1'  ini_sta=[1 0 0 0 0 0 0 0 0 0 0 0 1]  outBitMaskSource=Dialog parameter  shift=0  outVarSiz=off  maxOutSizeMode=Dialog parameter  maxOutSize=[10 1]  Ts=-1  sampPerFrame=1  reset=on  bitPackedOutputs=off  outDataType=boolean  numPackedBits=8  bitPackDataSigned=off  bitPackedOutDType=Smallest integer
  PN Sequence Generator12 : commseqgen3/PN Sequence Generator  poly='z^13 + z^12 + z^11 + z^8 + 1'  ini_sta=[1 0 0 1 0 0 0 0 0 1 0 0 1]  outBitMaskSource=Dialog parameter  shift=0  outVarSiz=off  maxOutSizeMode=Dialog parameter  maxOutSize=[10 1]  Ts=-1  sampPerFrame=1  reset=on  bitPackedOutputs=off  outDataType=boolean  numPackedBits=8  bitPackDataSigned=off  bitPackedOutDType=Smallest integer
  PN Sequence Generator13 : commseqgen3/PN Sequence Generator  poly='z^13 + z^12 + z^11 + z^8 + 1'  ini_sta=[1 1 1 1 1 1 0 1 1 1 1 1 1]  outBitMaskSource=Dialog parameter  shift=0  outVarSiz=off  maxOutSizeMode=Dialog parameter  maxOutSize=[10 1]  Ts=-1  sampPerFrame=1  reset=on  bitPackedOutputs=off  outDataType=boolean  numPackedBits=8  bitPackDataSigned=off  bitPackedOutDType=Smallest integer
  PN Sequence Generator14 : commseqgen3/PN Sequence Generator  poly='z^13 + z^12 + z^11 + z^8 + 1'  ini_sta=[1 0 1 0 1 0 1 0 1 0 1 0 1]  outBitMaskSource=Dialog parameter  shift=0  outVarSiz=off  maxOutSizeMode=Dialog parameter  maxOutSize=[10 1]  Ts=-1  sampPerFrame=1  reset=on  bitPackedOutputs=off  outDataType=boolean  numPackedBits=8  bitPackDataSigned=off  bitPackedOutDType=Smallest integer
  PN Sequence Generator15 : commseqgen3/PN Sequence Generator  poly='z^13 + z^12 + z^11 + z^8 + 1'  ini_sta=[0 1 0 1 0 1 0 1 0 1 0 1 0]  outBitMaskSource=Dialog parameter  shift=0  outVarSiz=off  maxOutSizeMode=Dialog parameter  maxOutSize=[10 1]  Ts=-1  sampPerFrame=1  reset=on  bitPackedOutputs=off  outDataType=boolean  numPackedBits=8  bitPackDataSigned=off  bitPackedOutDType=Smallest integer
  PN Sequence Generator16 : commseqgen3/PN Sequence Generator  poly='z^13 + z^12 + z^11 + z^8 + 1'  ini_sta=[1 1 1 0 0 0 1 1 1 0 0 0 1]  outBitMaskSource=Dialog parameter  shift=0  outVarSiz=off  maxOutSizeMode=Dialog parameter  maxOutSize=[10 1]  Ts=-1  sampPerFrame=1  reset=on  bitPackedOutputs=off  outDataType=boolean  numPackedBits=8  bitPackDataSigned=off  bitPackedOutDType=Smallest integer
  PN Sequence Generator17 : commseqgen3/PN Sequence Generator  poly='z^13 + z^12 + z^11 + z^8 + 1'  ini_sta=[0 0 0 0 0 1 1 0 0 0 1 1 1]  outBitMaskSource=Dialog parameter  shift=0  outVarSiz=off  maxOutSizeMode=Dialog parameter  maxOutSize=[10 1]  Ts=-1  sampPerFrame=1  reset=on  bitPackedOutputs=off  outDataType=boolean  numPackedBits=8  bitPackDataSigned=off  bitPackedOutDType=Smallest integer
  PN Sequence Generator18 : commseqgen3/PN Sequence Generator  poly='z^13 + z^12 + z^11 + z^8 + 1'  ini_sta=[1 1 0 0 0 1 1 1 1 0 0 0 0]  outBitMaskSource=Dialog parameter  shift=0  outVarSiz=off  maxOutSizeMode=Dialog parameter  maxOutSize=[10 1]  Ts=-1  sampPerFrame=1  reset=on  bitPackedOutputs=off  outDataType=boolean  numPackedBits=8  bitPackDataSigned=off  bitPackedOutDType=Smallest integer
  PN Sequence Generator19 : commseqgen3/PN Sequence Generator  poly='z^13 + z^12 + z^11 + z^8 + 1'  ini_sta=[1 1 1 1 1 1 1 0 0 0 0 0 0]  outBitMaskSource=Dialog parameter  shift=0  outVarSiz=off  maxOutSizeMode=Dialog parameter  maxOutSize=[10 1]  Ts=-1  sampPerFrame=1  reset=on  bitPackedOutputs=off  outDataType=boolean  numPackedBits=8  bitPackDataSigned=off  bitPackedOutDType=Smallest integer
  PN Sequence Generator2 : commseqgen3/PN Sequence Generator  poly='z^13 + z^12 + z^11 + z^8 + 1'  ini_sta=[1 1 0 1 0 0 0 0 0 1 0 0 1]  outBitMaskSource=Dialog parameter  shift=0  outVarSiz=off  maxOutSizeMode=Dialog parameter  maxOutSize=[10 1]  Ts=-1  sampPerFrame=1  reset=on  bitPackedOutputs=off  outDataType=boolean  numPackedBits=8  bitPackDataSigned=off  bitPackedOutDType=Smallest integer
  PN Sequence Generator3 : commseqgen3/PN Sequence Generator  poly='z^13 + z^12 + z^11 + z^8 + 1'  ini_sta=[1 0 1 0 0 0 0 1 0 0 1 1 0]  outBitMaskSource=Dialog parameter  shift=0  outVarSiz=off  maxOutSizeMode=Dialog parameter  maxOutSize=[10 1]  Ts=-1  sampPerFrame=1  reset=on  bitPackedOutputs=off  outDataType=boolean  numPackedBits=8  bitPackDataSigned=off  bitPackedOutDType=Smallest integer
  PN Sequence Generator4 : commseqgen3/PN Sequence Generator  poly='z^13 + z^12 + z^11 + z^8 + 1'  ini_sta=[0 0 0 0 1 0 0 0 0 1 1 1 0]  outBitMaskSource=Dialog parameter  shift=0  outVarSiz=off  maxOutSizeMode=Dialog parameter  maxOutSize=[10 1]  Ts=-1  sampPerFrame=1  reset=on  bitPackedOutputs=off  outDataType=boolean  numPackedBits=8  bitPackDataSigned=off  bitPackedOutDType=Smallest integer
  PN Sequence Generator5 : commseqgen3/PN Sequence Generator  poly='z^13 + z^12 + z^11 + z^8 + 1'  ini_sta=[1 1 0 0 1 1 0 0 1 0 1 0 0]  outBitMaskSource=Dialog parameter  shift=0  outVarSiz=off  maxOutSizeMode=Dialog parameter  maxOutSize=[10 1]  Ts=-1  sampPerFrame=1  reset=on  bitPackedOutputs=off  outDataType=boolean  numPackedBits=8  bitPackDataSigned=off  bitPackedOutDType=Smallest integer
  PN Sequence Generator6 : commseqgen3/PN Sequence Generator  poly='z^13 + z^12 + z^11 + z^8 + 1'  ini_sta=[1 0 0 0 0 1 0 0 0 0 1 1 1]  outBitMaskSource=Dialog parameter  shift=0  outVarSiz=off  maxOutSizeMode=Dialog parameter  maxOutSize=[10 1]  Ts=-1  sampPerFrame=1  reset=on  bitPackedOutputs=off  outDataType=boolean  numPackedBits=8  bitPackDataSigned=off  bitPackedOutDType=Smallest integer
  PN Sequence Generator7 : commseqgen3/PN Sequence Generator  poly='z^13 + z^12 + z^11 + z^8 + 1'  ini_sta=[1 0 0 1 1 1 1 1 0 0 0 1 1]  outBitMaskSource=Dialog parameter  shift=0  outVarSiz=off  maxOutSizeMode=Dialog parameter  maxOutSize=[10 1]  Ts=-1  sampPerFrame=1  reset=on  bitPackedOutputs=off  outDataType=boolean  numPackedBits=8  bitPackDataSigned=off  bitPackedOutDType=Smallest integer
  PN Sequence Generator8 : commseqgen3/PN Sequence Generator  poly='z^13 + z^12 + z^11 + z^8 + 1'  ini_sta=[1 1 0 1 1 1 1 1 0 0 0 1 1]  outBitMaskSource=Dialog parameter  shift=0  outVarSiz=off  maxOutSizeMode=Dialog parameter  maxOutSize=[10 1]  Ts=-1  sampPerFrame=1  reset=on  bitPackedOutputs=off  outDataType=boolean  numPackedBits=8  bitPackDataSigned=off  bitPackedOutDType=Smallest integer
  PN Sequence Generator9 : commseqgen3/PN Sequence Generator  poly='z^13 + z^12 + z^11 + z^8 + 1'  ini_sta=[0 1 0 1 1 0 0 1 0 0 0 1 1]  outBitMaskSource=Dialog parameter  shift=0  outVarSiz=off  maxOutSizeMode=Dialog parameter  maxOutSize=[10 1]  Ts=-1  sampPerFrame=1  reset=on  bitPackedOutputs=off  outDataType=boolean  numPackedBits=8  bitPackDataSigned=off  bitPackedOutDType=Smallest integer
  LFSR_G : Outport
  LFSR_F : Outport  Port=2
  wires:
  PN Sequence Generator/1 -> Bit Concat/1
  PN Sequence Generator3/1 -> Bit Concat/4
  PN Sequence Generator4/1 -> Bit Concat/5
  PN Sequence Generator1/1 -> Bit Concat/2
  PN Sequence Generator2/1 -> Bit Concat/3
  PN Sequence Generator5/1 -> Bit Concat/6
  PN Sequence Generator6/1 -> Bit Concat/7
  PN Sequence Generator7/1 -> Bit Concat/8
  PN Sequence Generator19/1 -> Bit Concat1/12
  PN Sequence Generator17/1 -> Bit Concat1/10
  PN Sequence Generator16/1 -> Bit Concat1/9
  PN Sequence Generator15/1 -> Bit Concat1/8
  PN Sequence Generator12/1 -> Bit Concat1/5
  PN Sequence Generator14/1 -> Bit Concat1/7
  PN Sequence Generator13/1 -> Bit Concat1/6
  PN Sequence Generator18/1 -> Bit Concat1/11
  Reset/1 -> PN Sequence Generator1/1, PN Sequence Generator4/1, PN Sequence Generator5/1, PN Sequence Generator6/1, PN Sequence Generator7/1, PN Sequence Generator10/1, PN Sequence Generator12/1, PN Sequence Generator13/1, PN Sequence Generator14/1, PN Sequence Generator15/1, PN Sequence Generator16/1, PN Sequence Generator17/1, PN Sequence Generator19/1, PN Sequence Generator18/1, PN Sequence Generator11/1, PN Sequence Generator9/1, PN Sequence Generator8/1, PN Sequence Generator3/1, PN Sequence Generator2/1, PN Sequence Generator/1
  Bit Concat/1 -> LFSR_G/1
  Bit Concat1/1 -> LFSR_F/1
  PN Sequence Generator8/1 -> Bit Concat1/1
  PN Sequence Generator9/1 -> Bit Concat1/2
  PN Sequence Generator10/1 -> Bit Concat1/3
  PN Sequence Generator11/1 -> Bit Concat1/4

== system fec_ber_hw/AWGN Channel/sample_and_hold/tvalid hold ==
  In1 : Inport
  Compare To Constant : simulink/Logic and Bit Operations/Compare To Constant  relop===  const=7  OutDataTypeStr=boolean
  Delay1 : Delay  DelayLength=1
  HDL Counter : hdlsllib/Sources/HDL Counter  CountType=Count limited  CountInit=0  CountStep=1  CountMax=7  CountFromType=Initial value  CountFrom=0  CountResetPort=off  CountLoadPort=off  CountEnbPort=on  CountDirPort=off  CountDataType=Unsigned  CountWordLen=3  CountFracLen=0  CountSampTime=1
  OR : Logic  Operator=OR  IconShape=distinctive  AllPortsSameDT=off  OutDataTypeStr=boolean
  Sample and Hold1 : dspsigops/Sample and Hold  trig=Rising edge  initCond=0  latchinput=off
  " " : Outport
  wires:
  In1/1 -> OR/2, Sample and Hold1/1
  Sample and Hold1/1 -> HDL Counter/1, " "/1
  Compare To Constant/1 -> Delay1/1
  OR/1 -> Sample and Hold1/Trigger
  Delay1/1 -> OR/1
  HDL Counter/1 -> Compare To Constant/1

== system fec_ber_hw/Encoder/sample_and_hold/tvalid hold ==
  In1 : Inport
  Compare To Constant : simulink/Logic and Bit Operations/Compare To Constant  relop===  const=3  OutDataTypeStr=boolean
  HDL Counter : hdlsllib/Sources/HDL Counter  CountType=Count limited  CountInit=0  CountStep=1  CountMax=7  CountFromType=Initial value  CountFrom=0  CountResetPort=on  CountLoadPort=off  CountEnbPort=on  CountDirPort=off  CountDataType=Unsigned  CountWordLen=3  CountFracLen=0  CountSampTime=1
  OR : Logic  Operator=OR  IconShape=distinctive  AllPortsSameDT=off  OutDataTypeStr=boolean
  Sample and Hold1 : dspsigops/Sample and Hold  trig=Rising edge  initCond=0  latchinput=off
  " " : Outport
  wires:
  In1/1 -> OR/2, Sample and Hold1/1
  Sample and Hold1/1 -> HDL Counter/2, " "/1
  OR/1 -> HDL Counter/1, Sample and Hold1/Trigger
  Compare To Constant/1 -> OR/1
  HDL Counter/1 -> Compare To Constant/1
